simulink model "gps_simplehost_demo"  (Simulink 7.3)
settings: Solver=FixedStepDiscrete  SolverMode=SingleTasking  StartTime=0.0  StopTime=inf  RelTol=1e-3
libraries: rapidstm32_addon_lib x1
settings Model: Creator=Compaq  LastModifiedBy=Krisada
settings OptimizationCC: StateBitsets=on  DataBitsets=on  UseTempVars=on  ZeroExternalMemoryAtStartup=off  ZeroInternalMemoryAtStartup=off  OptimizeModelRefInitCode=on  LifeSpan=1
settings HardwareCC: ProdEndianess=LittleEndian  ProdHWDeviceType=ARM Compatible->Cortex - M3  TargetEndianess=LittleEndian  TargetHWDeviceType=ARM Compatible->Cortex - M3
settings RTWCC: SystemTargetFile=rapidstm32.tlc  GenerateMakefile=off  TemplateMakefile=rapidstm32_rvmdk.tmf  Description=Rapid STM32 Target  GenerateReport=on  RetainRTWFile=on  ProcessScript=rapidstm32_make_rtw_hook  IncludeHyperlinkInReport=on
settings CodeAppCC: IgnoreCustomStorageClasses=off
settings STFCustomTargetCC: ModelReferenceCompliant=off  CombineOutputUpdateFcns=on  ERTCustomFileBanners=on  SupportContinuousTime=off  SupportNonInlinedSFcns=off  SystemTargetFile=rapidstm32.tlc
settings ERTTargetCC: MultiwordLength=2048  ModelReferenceCompliant=off  ParMdlRefBuildCompliant=off  CompOptLevelCompliant=off  ERTFirstTimeCompliant=off  ModelStepFunctionPrototypeControlCompliant=off  CPPClassGenCompliant=off  ExtModeMexFile=ext_rapidstm32_serial_win32  InlinedParameterPlacement=NonHierarchical  ERTSrcFileBannerTemplate=rapidstm32_code_template.cgt  ERTHdrFileBannerTemplate=rapidstm32_code_template.cgt  ERTDataSrcFileTemplate=rapidstm32_code_template.cgt  ERTDataHdrFileTemplate=rapidstm32_code_template.cgt  ERTCustomFileTemplate=rapidstm32_file_process.tlc
settings CustomProperty: DataType=RTWOptions_EnumType_C__rapidstm32_rapidstm32_rapidstm32_1RapidSTM32Board  Value=FiO Std
settings EnumStrPairs: String=FiO Std

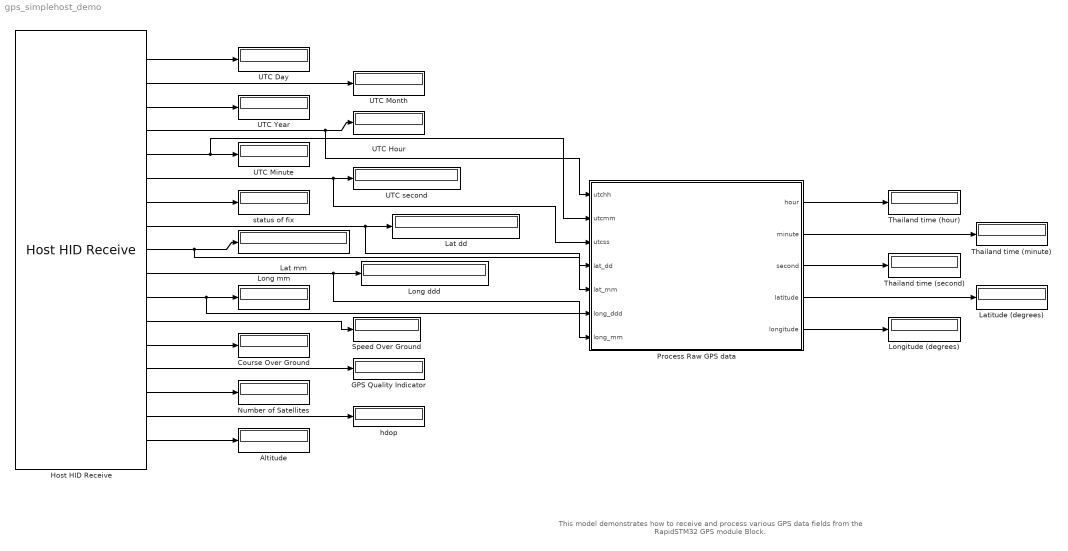
== system gps_simplehost_demo ==
  note: This model demonstrates how to receive and process various GPS data fields from the RapidSTM32 GPS module Block.
  Altitude : Display
  Course Over Ground : Display
  GPS Quality Indicator : Display
  Host HID Receive : rapidstm32_addon_lib/Host HID Receive  Priority=1  binformat='uint8 uint8 uint8 uint8 uint8 uint16 uint8 int16 uint32 int16 uint32 single single uint8 uint8 single single'  sampletime=1  blocking=on  output_nonblocking=Zeros  timeout=10  read_elapse_msec=off
  Lat dd : Display
  Lat mm : Display
  Latitude (degrees) : Display
  Long ddd : Display
  Long mm : Display
  Longitude (degrees) : Display
  Number of Satellites : Display
  Process Raw GPS data : Stateflow chart
  Speed Over Ground : Display
  Thailand time (hour) : Display
  Thailand time (minute) : Display
  Thailand time (second) : Display
  UTC Day : Display
  UTC Hour : Display
  UTC Minute : Display
  UTC Month : Display
  UTC Year : Display
  UTC second : Display
  hdop : Display
  status of fix : Display
  wires:
  Host HID Receive/1 -> UTC Day/1
  Host HID Receive/2 -> UTC Month/1
  Host HID Receive/3 -> UTC Year/1
  Host HID Receive/4 -> UTC Hour/1, Process Raw GPS data/1(utchh)
  Host HID Receive/5 -> UTC Minute/1, Process Raw GPS data/2(utcmm)
  Host HID Receive/6 -> UTC second/1, Process Raw GPS data/3(utcss)
  Host HID Receive/7 -> status of fix/1
  Host HID Receive/8 -> Lat dd/1, Process Raw GPS data/4(lat_dd)
  Host HID Receive/9 -> Lat mm/1, Process Raw GPS data/5(lat_mm)
  Host HID Receive/10 -> Long ddd/1, Process Raw GPS data/6(long_ddd)
  Host HID Receive/11 -> Long mm/1, Process Raw GPS data/7(long_mm)
  Host HID Receive/12 -> Speed Over Ground/1
  Host HID Receive/13 -> Course Over Ground/1
  Host HID Receive/14 -> GPS Quality Indicator/1
  Host HID Receive/15 -> Number of Satellites/1
  Host HID Receive/16 -> hdop/1
  Host HID Receive/17 -> Altitude/1
  Process Raw GPS data/1(hour) -> Thailand time (hour)/1
  Process Raw GPS data/2(minute) -> Thailand time (minute)/1
  Process Raw GPS data/3(second) -> Thailand time (second)/1
  Process Raw GPS data/4(latitude) -> Latitude (degrees)/1
  Process Raw GPS data/5(longitude) -> Longitude (degrees)/1

== matlab function Process Raw GPS data ==
  data: utchh input double; utcmm input double; utcss input double; hour output double; minute output double; second output double; lat_dd input double; latitude output double; lat_mm input double; long_ddd input double; long_mm input double; longitude output double
function [hour, minute, second, latitude, longitude] = ProcessRawGPSData(utchh, utcmm, utcss, lat_dd, lat_mm, long_ddd, long_mm)
%#eml

% Input
% utchh, utcmm, utcss, lat_dd, lat_mm, long_ddd, long_mm from GPS Module Block
%
% Output
% hour, minute, second in Thailand time (GMT + 7)
% latitude and longitude are in degrees

hour = utchh + 7;
minute = utcmm;
second = single(utcss)/1000;
latitude = single(lat_dd) + ((single(lat_mm) / (10^6)) / 60);
longitude = single(long_ddd) + ((single(long_mm) / (10^6)) / 60);
